simulink model "PID_2015"  (Simulink 8.5)
settings: Solver=ode5  StartTime=0.0  StopTime=tf+1  FixedStep=0.005  RelTol=1e-3  AbsTol=1e-6
values from neighbouring files (symbols this model uses):
  Kd = 3*a.*omega - Fv    [init_PID.m]
  Ki = a.*omega.^3    [init_PID.m]
  Kp = 6*a.*omega.^2    [init_PID.m]    (also in init_torque.m = omega.^2)
  kt = [20 7]    [init_PID.m]    (also in init_torque.m)
  ListePoints = [100*pi/360 100*pi/360;6*pi/360 60*pi/360]    [init_PID.m]    (also in init_torque.m)
undefined symbols (not defined in the file or in its folder): inter_arti_d5, scarabase_ddm
settings Model: Creator=user  LastModifiedBy=steff  ExtModeTrigMode=oneshot  ExtModeArmWhenConnect=off
settings DataIOCC: LimitDataPoints=off  SignalLoggingName=sigsOut
settings OptimizationCC: BooleanDataType=off
settings DebuggingCC: SaveWithParameterizedLinksMsg=none  SignalResolutionControl=TryResolveAllWithWarning  MultiTaskDSMMsg=warning  MultiTaskCondExecSysMsg=none  FcnCallInpInsideContextMsg=EnableAllAsError
settings HardwareCC: TargetUnknown=on
settings RTWCC: TemplateMakefile=grt_vc.tmf

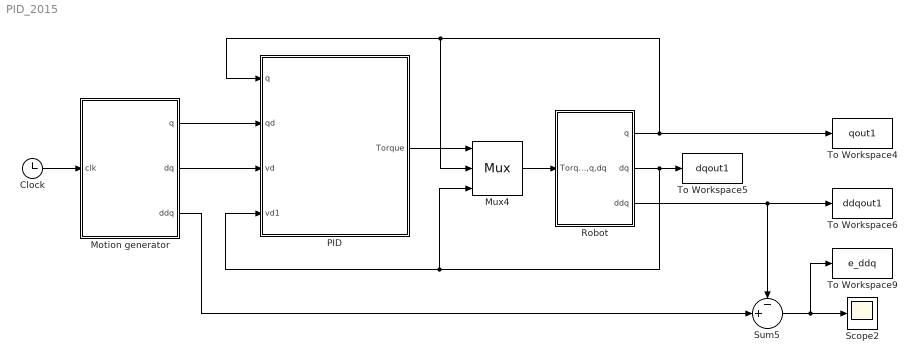
== system PID_2015 ==
  Clock : Clock
  Motion generator : Subsystem
  Mux4 : Mux  Inputs=3
  PID : Subsystem
  Robot : Subsystem
  Scope2 : Scope
      settings: TimeRange=auto  LimitDataPoints=on  MaxDataPoints=5000  SaveToWorkspace=off  SaveName=ScopeData  YMin=-10  YMax=10  SampleTime=-1  DataFormat=Array
  Sum5 : Sum  Inputs=-+|
  To Workspace4 : ToWorkspace  VariableName=qout1  SampleTime=-1
  To Workspace5 : ToWorkspace  VariableName=dqout1  SampleTime=-1
  To Workspace6 : ToWorkspace  VariableName=ddqout1  SampleTime=-1
  To Workspace9 : ToWorkspace  VariableName=e_ddq  SampleTime=-1
  wires:
  Sum5/1 -> To Workspace9/1, Scope2/1
  Motion generator/3(ddq) -> Sum5/2
  Clock/1 -> Motion generator/1(clk)
  Robot/3(ddq) -> Sum5/1, To Workspace6/1
  Robot/2(dq) -> PID/4(vd1), Mux4/3, To Workspace5/1
  Mux4/1 -> Robot/1(Torque,q,dq)
  Robot/1(q) -> Mux4/2, PID/1("q "), To Workspace4/1
  Motion generator/1(q) -> PID/2(qd)
  Motion generator/2(dq) -> PID/3(vd)
  PID/1(Torque) -> Mux4/1

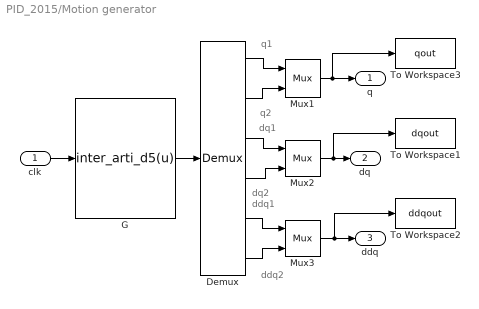
== system PID_2015/Motion generator ==
  note: q1
  note: q2
  note: dq1
  note: dq2
  note: ddq1
  note: ddq2
  clk : Inport
  Demux : Demux  Outputs=6
  G : MATLABFcn  MATLABFcn=inter_arti_d5(u)  OutputDimensions=6  Output1D=off
  Mux1 : Mux  Inputs=2
  Mux2 : Mux  Inputs=2
  Mux3 : Mux  Inputs=2
  To Workspace1 : ToWorkspace  VariableName=dqout  SampleTime=-1
  To Workspace2 : ToWorkspace  VariableName=ddqout  SampleTime=-1
  To Workspace3 : ToWorkspace  VariableName=qout  SampleTime=-1
  q : Outport
  dq : Outport  Port=2
  ddq : Outport  Port=3
  wires:
  Demux/6 -> Mux3/2
  Demux/5 -> Mux3/1
  Demux/1 -> Mux1/1
  Demux/4 -> Mux2/2
  clk/1 -> G/1
  Demux/3 -> Mux2/1
  G/1 -> Demux/1
  Demux/2 -> Mux1/2
  Mux1/1 -> To Workspace3/1, q/1
  Mux3/1 -> To Workspace2/1, ddq/1
  Mux2/1 -> To Workspace1/1, dq/1

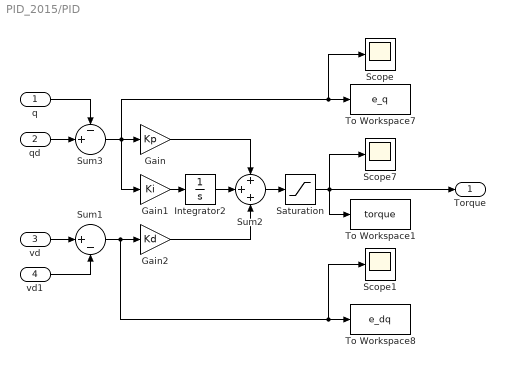
== system PID_2015/PID ==
  "q " : Inport
  qd : Inport  Port=2
  vd : Inport  Port=3
  vd1 : Inport  Port=4
  Gain : Gain  Gain=Kp
  Gain1 : Gain  Gain=Ki
  Gain2 : Gain  Gain=Kd
  Integrator2 : Integrator  InitialCondition=[0 0]
  Saturation : Saturate  UpperLimit=kt  LowerLimit=-kt
  Scope : Scope
      settings: TimeRange=auto  LimitDataPoints=on  MaxDataPoints=5000  SaveToWorkspace=off  SaveName=ScopeData  YMin=-0.00446  YMax=0.00509  SampleTime=-1
  Scope1 : Scope
      settings: TimeRange=auto  LimitDataPoints=on  MaxDataPoints=5000  SaveToWorkspace=off  SaveName=ScopeData  YMin=-10  YMax=10  SampleTime=-1  DataFormat=Array
  Scope7 : Scope
      settings: TimeRange=auto  LimitDataPoints=on  MaxDataPoints=5000  SaveToWorkspace=off  SaveName=ScopeData7  YMin=-21.20919  YMax=21.76654  SampleTime=-1
  Sum1 : Sum  Inputs=|+-
  Sum2 : Sum  Inputs=+++
  Sum3 : Sum  Inputs=-+|
  To Workspace1 : ToWorkspace  VariableName=torque  SampleTime=-1
  To Workspace7 : ToWorkspace  VariableName=e_q  SampleTime=-1
  To Workspace8 : ToWorkspace  VariableName=e_dq  SampleTime=-1
  Torque : Outport
  wires:
  qd/1 -> Sum3/2
  Gain2/1 -> Sum2/3
  Sum2/1 -> Saturation/1
  Sum3/1 -> To Workspace7/1, Scope/1, Gain1/1, Gain/1
  Sum1/1 -> To Workspace8/1, Scope1/1, Gain2/1
  Gain1/1 -> Integrator2/1
  Saturation/1 -> To Workspace1/1, Scope7/1, Torque/1
  Integrator2/1 -> Sum2/2
  Gain/1 -> Sum2/1
  vd/1 -> Sum1/1
  "q "/1 -> Sum3/1
  vd1/1 -> Sum1/2

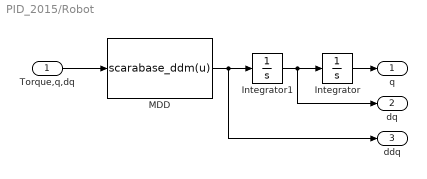
== system PID_2015/Robot ==
  Torque,q,dq : Inport
  Integrator : Integrator  InitialCondition=ListePoints(1,:)
  Integrator1 : Integrator  InitialCondition=[0 0]
  MDD : MATLABFcn  MATLABFcn=scarabase_ddm(u)  OutputDimensions=2
  q : Outport
  dq : Outport  Port=2
  ddq : Outport  Port=3
  wires:
  Integrator/1 -> q/1
  MDD/1 -> ddq/1, Integrator1/1
  Integrator1/1 -> dq/1, Integrator/1
  Torque,q,dq/1 -> MDD/1
